simulink model "P2_simulinkModel"  (R2024b)
settings: Solver=VariableStepAuto  StartTime=0.0  StopTime=1  RelTol=1e-3
libraries: sdrrlib x1
settings Model: Creator=javit  LastModifiedBy=javit

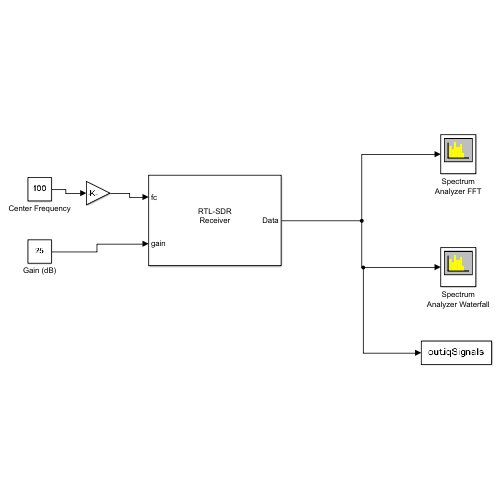
[thumbnail: Simulink's stored preview of the top-level diagram]
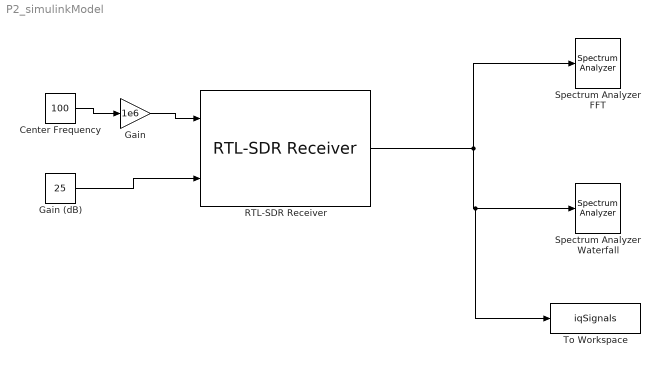
== system P2_simulinkModel ==
  Center Frequency : Constant  Value=100
  Gain : Gain  Gain=1e6
  Gain (dB) : Constant  Value=25
  RTL-SDR Receiver : sdrrlib/RTL-SDR Receiver  IPAddress=0  CenterFrequencySource=Input port  CenterFrequency=102.5e6  GainSource=Input port  Gain=0  ADCRate=2.4e6  FrequencyCorrection=0  LostSamplesOutputPort=off  LatencyOutputPort=off  OutputDataType=single  FrameLength=4096  EnableBurstMode=off  NumFramesInBurst=20  sobjType=sdrr.internal.SDRRTLReceiverSL  dataUDPPort=-1  ctrlUDPPort=-1  subDeviceList=nosubdev  sdrBlockType=SDRBlockTypeSLT.SDRRxBlock  requester=UNUSED_BY_SFCN  sdrExecutionMode=SDRExecutionModeSLT.ExecModeHW  BypassUserLogic=off  DecimatorSelect=DDC decimator  SourceSelect=RF data  SineAmplitude=16000  EnableInternalClock=off  BypassIQBalance=off  IFBandwidth=40e6  ADCRateSource=Dialog  IntermediateFrequency=0  DecimationFactorSource=Dialog  DecimationFactor=512  RFFrequencyIsTunable=logical(1)  SampleTime=(4096)/(2.4e6)  IFBandwidthSource=Dialog  SineFrequency=30000  BypassDCBlockingFilter=off  IntermediateFrequencySource=Dialog  IQBalanceCoefficients=64  SkipAllHardwareResetAndInitialization=off  EnableIQCalibrationTable=on  CacheIQCalibrationTable=off  EnableOffsetTuning=off  EnableRTLAGC=off  EnableTestMode=off  EnableTunerAGC=off  FrequencyCorrectionSource=Dialog  NumMLBuffers=128  NumUSBBuffers=16  RTLCrystalFrequency=28800000  TunerCrystalFrequency=28800000
  Spectrum Analyzer FFT : SpectrumAnalyzer  WindowPosition=[2597.000000,142.000000,800.000000,500.000000,]  Visible=on  ScopeFrameLocation=window  WindowInvariantSamplesPerUpdate=on  Span=2400000  StartFrequency=-1200000  StopFrequency=1200000  YLimits=[-39.88687557,14.65027788]
  Spectrum Analyzer Waterfall : SpectrumAnalyzer  WindowPosition=[681.000000,105.000000,800.000000,500.000000,]  Visible=on  ScopeFrameLocation=window  ViewType=Spectrogram  WindowInvariantSamplesPerUpdate=on  Span=2400000  StartFrequency=-1200000  StopFrequency=1200000  ReferenceLoad=50  ColorLimits=[-58.66969123,-1.85145325]
  To Workspace : ToWorkspace  VariableName=iqSignals  SaveFormat=Structure With Time  SampleTime=-1
  wires:
  Gain (dB)/1 -> RTL-SDR Receiver/2
  Center Frequency/1 -> Gain/1
  Gain/1 -> RTL-SDR Receiver/1
  RTL-SDR Receiver/1 -> To Workspace/1, Spectrum Analyzer Waterfall/1, Spectrum Analyzer FFT/1
